simulink model "OTSG_v1"  (R2018a)
settings: Solver=ode23tb  StartTime=0.0  StopTime=2500  MaxStep=0.1  RelTol=1e-3
values from neighbouring files (symbols this model uses):
  A_s = 1.2245    [MSDR_parameters.m]
  Cp_p = 5763.597e-6    (= 0.005763597)    [MSDR_parameters.m]
  Cp_s = 3588.208e-6    (= 0.003588208)    [MSDR_parameters.m]
  Cp_sc = 4761.392e-6    (= 0.004761392)    [MSDR_parameters.m]
  Cp_w = 456.056e-6    (= 0.000456056)    [MSDR_parameters.m]
  D_it = 0.0141478    [MSDR_parameters.m]
  D_ot = 0.015875    [MSDR_parameters.m]
  dHs_dPs = -0.042433622114357    (= -0.0424336221144)    [MSDR_parameters.m]
  h_pw = 9101.343578935E-6    (= 0.00910134357894)    [MSDR_parameters.m]
  h_wb = 13349.334646671E-6    (= 0.0133493346467)    [MSDR_parameters.m]
  h_ws = 5732.378387768E-6    (= 0.00573237838777)    [MSDR_parameters.m]
  h_wsc = 8385.005556375E-6    (= 0.00838500555638)    [MSDR_parameters.m]
  K_1 = 11.632248097704855    (= 11.6322480977)    [MSDR_parameters.m]
  K_b = 12.834854076292217    (= 12.8348540763)    [MSDR_parameters.m]
  K_sc = -17.615718797133468    (= -17.6157187971)    [MSDR_parameters.m]
  L = 8.5344    [MSDR_parameters.m]
  L_b = 5.97408    [MSDR_parameters.m]
  L_s = 1.28016    [MSDR_parameters.m]
  M_stm = 0.018    [MSDR_parameters.m]
  N = 6546    [MSDR_parameters.m]
  P_s = 5.8    [MSDR_parameters.m]
  P_sat = 6    [MSDR_parameters.m]
  P_sc = 5.8    [MSDR_parameters.m]
  P_set = 5.8    [MSDR_parameters.m]
  R = 8.314462E-6    (= 8.314462e-06)    [MSDR_parameters.m]
  rho_p = 716.826    [MSDR_parameters.m]
  rho_s = 26.5561    [MSDR_parameters.m]
  rho_sc = (rho_fw + rho_f)/2    (= 789.7745)    [MSDR_parameters.m]
  rho_w = 8425.712    [MSDR_parameters.m]
  T_p1 = 320.712    [MSDR_parameters.m]
  T_p2 = 320.478    [MSDR_parameters.m]
  T_p3 = 311.033    [MSDR_parameters.m]
  T_p4 = 305.206    [MSDR_parameters.m]
  T_p5 = 303.289    [MSDR_parameters.m]
  T_p6 = 297.506    [MSDR_parameters.m]
  T_s1 = 313.717    [MSDR_parameters.m]
  T_s2 = 307.462    [MSDR_parameters.m]
  T_sc1 = 274.967    [MSDR_parameters.m]
  T_w1 = 320.344    [MSDR_parameters.m]
  T_w2 = 319.794    [MSDR_parameters.m]
  T_w3 = 301.311    [MSDR_parameters.m]
  T_w4 = 299.206    [MSDR_parameters.m]
  T_w5 = 298.512    [MSDR_parameters.m]
  T_w6 = 283.112    [MSDR_parameters.m]
  W_fw = 226.7962    [MSDR_parameters.m]
  W_p0 = 3779.937    [MSDR_parameters.m]
  Z_ss = 0.76634    [MSDR_parameters.m]
settings Model: Creator=viikr  LastModifiedBy=Vikram Singh
settings SolverCC: AlgebraicLoopSolver=LineSearch

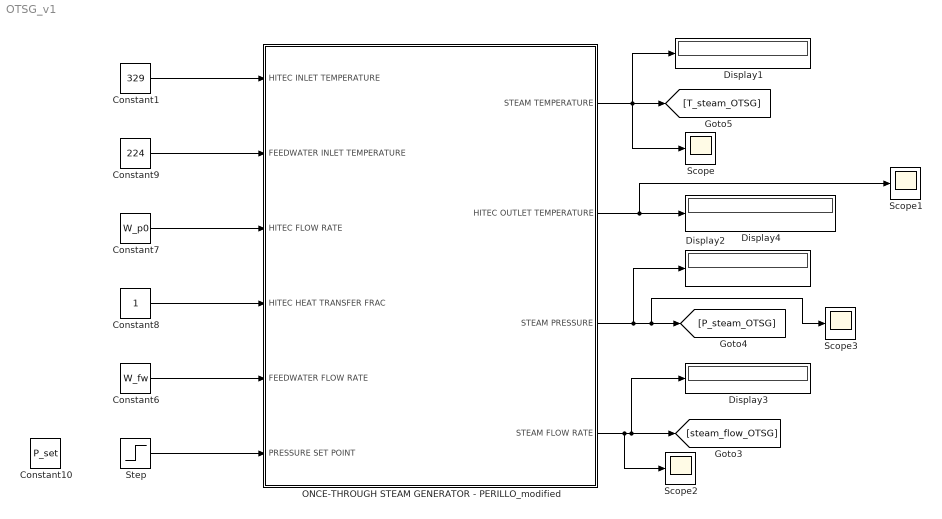
== system OTSG_v1 ==
  Constant1 : Constant  Value=329
  Constant10 : Constant  Value=P_set
  Constant6 : Constant  Value=W_fw
  Constant7 : Constant  Value=W_p0
  Constant8 : Constant
  Constant9 : Constant  Value=224
  Display{1..4} (4 alike) : Display
  ONCE-THROUGH STEAM GENERATOR - PERILLO_modified : Subsystem
  Scope{,1..3} (4 alike) : Scope
  Step : Step  Time=1000  Before=5.8  After=5.9  SampleTime=0
  wires:
  Constant9/1 -> ONCE-THROUGH STEAM GENERATOR - PERILLO_modified/2(FEEDWATER INLET TEMPERATURE)
  ONCE-THROUGH STEAM GENERATOR - PERILLO_modified/1(STEAM TEMPERATURE) -> Scope/1, Display1/1, [T_steam_OTSG]
  Constant8/1 -> ONCE-THROUGH STEAM GENERATOR - PERILLO_modified/4(HITEC HEAT TRANSFER FRAC)
  ONCE-THROUGH STEAM GENERATOR - PERILLO_modified/2(HITEC OUTLET TEMPERATURE) -> Scope1/1, Display4/1
  Constant7/1 -> ONCE-THROUGH STEAM GENERATOR - PERILLO_modified/3(HITEC FLOW RATE)
  ONCE-THROUGH STEAM GENERATOR - PERILLO_modified/4(STEAM FLOW RATE) -> Scope2/1, [steam_flow_OTSG], Display3/1
  ONCE-THROUGH STEAM GENERATOR - PERILLO_modified/3(STEAM PRESSURE) -> Scope3/1, [P_steam_OTSG], Display2/1
  Constant6/1 -> ONCE-THROUGH STEAM GENERATOR - PERILLO_modified/5(FEEDWATER FLOW RATE)
  Constant1/1 -> ONCE-THROUGH STEAM GENERATOR - PERILLO_modified/1(HITEC INLET TEMPERATURE)
  Step/1 -> ONCE-THROUGH STEAM GENERATOR - PERILLO_modified/6(PRESSURE SET POINT)

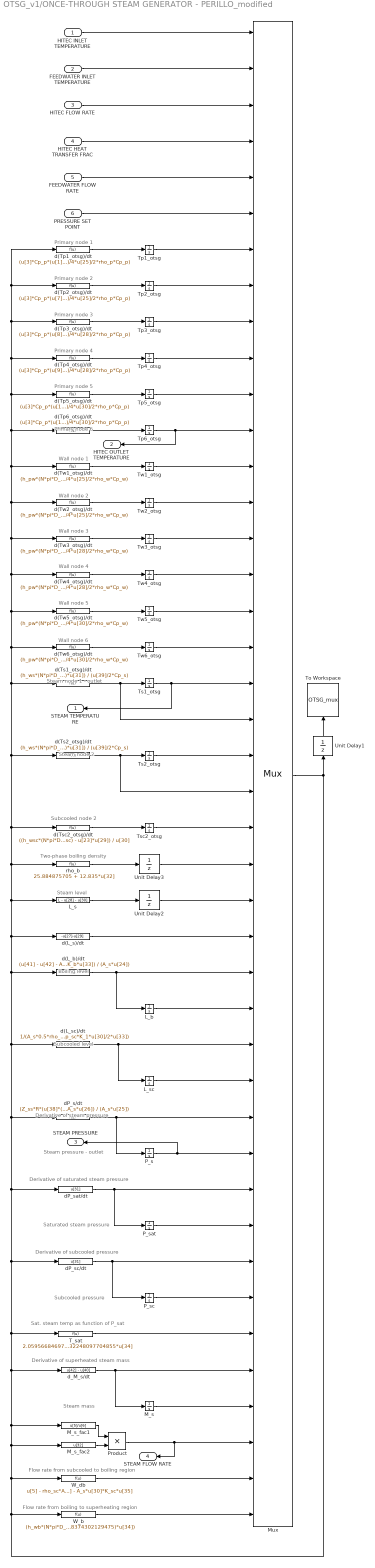
== system OTSG_v1/ONCE-THROUGH STEAM GENERATOR - PERILLO_modified ==
  note: Primary node 1
  note: Primary node 2
  note: Primary node 3
  note: Primary node 4
  note: Primary node 5
  note: Primary node 6
  note: Wall node 1
  note: Wall node 2
  note: Wall node 3
  note: Wall node 4
  note: Wall node 5
  note: Wall node 6
  note: Steam node 1 - outlet
  note: Steam level
  note: Boiling level
  note: Subcooled level
  note: Derivative of saturated steam pressure
  note: Sat. steam temp as function of P_sat
  note: Saturated steam pressure
  note: Subcooled pressure
  note: Derivative of steam pressure
  note: Derivative of subcooled pressure
  note: Steam pressure - outlet
  note: Subcooled node 2
  note: Steam node 2
  note: Two-phase boiling density
  note: Derivative of superheated steam mass
  note: Steam mass
  note: Flow rate from subcooled to boiling region
  note: Flow rate from boiling to superheating region
  HITEC INLET TEMPERATURE : Inport
  FEEDWATER INLET TEMPERATURE : Inport  Port=2
  HITEC FLOW RATE : Inport  Port=3
  HITEC HEAT TRANSFER FRAC : Inport  Port=4
  FEEDWATER FLOW RATE : Inport  Port=5
  PRESSURE SET POINT : Inport  Port=6
  L_b : Integrator  InitialCondition=L_b
  L_s : Fcn  Expr=L - u[28] - u[30]
  L_sc : Integrator  InitialCondition=.5344
  M_s : Integrator  InitialCondition=rho_s*A_s*L_s
  M_s_fac1 : Fcn  Expr=u[5]/u[6]
  M_s_fac2 : Fcn  Expr=u[32]
  Mux : Mux  Inputs=42
      settings: DisplayOption=signals
  P_s : Integrator  InitialCondition=P_s
  P_sat : Integrator  InitialCondition=P_sat
  P_sc : Integrator  InitialCondition=P_sc
  Product : Product
  T_sat : Fcn  Expr=2.059566846979075e+02 + 11.632248097704855*u[34]
  To Workspace : ToWorkspace  VariableName=OTSG_mux  SampleTime=-1
      settings: Save2DSignal=2-D array (concatenate along first dimension)
  Tp1_otsg : Integrator  InitialCondition=T_p1
  Tp2_otsg : Integrator  InitialCondition=T_p2
  Tp3_otsg : Integrator  InitialCondition=T_p3
  Tp4_otsg : Integrator  InitialCondition=T_p4
  Tp5_otsg : Integrator  InitialCondition=T_p5
  Tp6_otsg : Integrator  InitialCondition=T_p6
  Ts1_otsg : Integrator  InitialCondition=T_s1
  Ts2_otsg : Integrator  InitialCondition=T_s2
  Tsc2_otsg : Integrator  InitialCondition=T_sc1
  Tw1_otsg : Integrator  InitialCondition=T_w1
  Tw2_otsg : Integrator  InitialCondition=T_w2
  Tw3_otsg : Integrator  InitialCondition=T_w3
  Tw4_otsg : Integrator  InitialCondition=T_w4
  Tw5_otsg : Integrator  InitialCondition=T_w5
  Tw6_otsg : Integrator  InitialCondition=T_w6
  Unit Delay1 : UnitDelay  SampleTime=-1
  Unit Delay2 : UnitDelay  InitialCondition=L_s  SampleTime=-1
  Unit Delay3 : UnitDelay  InitialCondition=100.307656893  SampleTime=-1
  W_b : Fcn  Expr=(h_wb*(N*pi*D_ot*u[28])*(0.5*u[15] + 0.5*u[16] - u[37])) / (1.980883222760319 + (-0.068374302129475)*u[34])
  W_db : Fcn  Expr=u[5] - rho_sc*A_s*u[29] - A_s*u[30]*K_sc*u[35]
  d(L_b)/dt : Fcn  Expr=(u[41] - u[42] - A_s*u[28]*K_b*u[33]) / (A_s*u[24])
  d(L_s)/dt : Fcn  Expr=-u[27]-u[29]
  d(L_sc)/dt : Fcn  Expr=1/(A_s*0.5*rho_sc*Cp_sc*(u[23] - u[37])) * (h_wsc*N*pi*D_ot*u[30]/2*(u[17] - u[37]) + u[5]*Cp_sc*(u[23] - u[37]) - A_s*u[30]/2*(K_sc*Cp_sc*(u[23] - 2*u[37]) - 1)*u[35] - A_s*rho_sc*Cp_sc*K_1*u[30]/2*u[33])
  d(Tp1_otsg)/dt : Fcn  Expr=(u[3]*Cp_p*(u[1] - u[7]) + h_pw*(N*pi*D_it*u[25]/2)*(u[13] - u[7])) / (N*pi*(D_it^2)/4*u[25]/2*rho_p*Cp_p)
  d(Tp2_otsg)/dt : Fcn  Expr=(u[3]*Cp_p*(u[7] - u[8]) + h_pw*(N*pi*D_it*u[25]/2)*(u[14] - u[8])) / (N*pi*(D_it^2)/4*u[25]/2*rho_p*Cp_p)
  d(Tp3_otsg)/dt : Fcn  Expr=(u[3]*Cp_p*(u[8] - u[9]) + h_pw*(N*pi*D_it*u[28]/2)*(u[15] - u[9])) / (N*pi*(D_it^2)/4*u[28]/2*rho_p*Cp_p)
  d(Tp4_otsg)/dt : Fcn  Expr=(u[3]*Cp_p*(u[9] - u[10]) + h_pw*(N*pi*D_it*u[28]/2)*(u[16] - u[10])) / (N*pi*(D_it^2)/4*u[28]/2*rho_p*Cp_p)
  d(Tp5_otsg)/dt : Fcn  Expr=(u[3]*Cp_p*(u[10] - u[11]) + h_pw*(N*pi*D_it*u[30]/2)*(u[17] - u[11])) / (N*pi*(D_it^2)/4*u[30]/2*rho_p*Cp_p)
  d(Tp6_otsg)/dt : Fcn  Expr=(u[3]*Cp_p*(u[11] - u[12]) + h_pw*(N*pi*D_it*u[30]/2)*(u[18] - u[12])) / (N*pi*(D_it^2)/4*u[30]/2*rho_p*Cp_p)
  d(Ts1_otsg)/dt : Fcn  Expr=(h_ws*(N*pi*D_ot*u[25]/2)*(u[13] - u[19]) + u[40]*Cp_s*(u[21] - u[19]) + Cp_s*(u[21] - u[19])*u[38]/2 + (A_s*u[25]/2 - u[39]/2*dHs_dPs)*u[31]) / (u[39]/2*Cp_s)
  d(Ts2_otsg)/dt : Fcn  Expr=(h_ws*(N*pi*D_ot*u[25]/2)*(u[14] - u[21]) + u[42]*Cp_s*(u[37] - u[21]) + (A_s*u[25]/2 - u[39]/2*dHs_dPs)*u[31]) / (u[39]/2*Cp_s)
  d(Tsc2_otsg)/dt : Fcn  Expr=((h_wsc*(N*pi*D_ot*u[30]/2)*(u[18] - u[23]) + Cp_sc*(u[5]*u[2] - (u[5] + u[41])*0.5*u[23]) + A_s*u[30]/2*u[35]) * 2/(A_s*rho_sc*Cp_sc) - u[23]*u[29]) / u[30]
  d(Tw1_otsg)/dt : Fcn  Expr=(h_pw*(N*pi*D_it*u[25]/2)*(u[7] - u[13]) + h_ws*(N*pi*D_ot*u[25]/2)*(u[19] - u[13])) / (N*pi*(D_ot^2 - D_it^2)/4*u[25]/2*rho_w*Cp_w)
  d(Tw2_otsg)/dt : Fcn  Expr=(h_pw*(N*pi*D_it*u[25]/2)*(u[8] - u[14]) + h_ws*(N*pi*D_ot*u[25]/2)*(u[21] - u[14])) / (N*pi*(D_ot^2 - D_it^2)/4*u[25]/2*rho_w*Cp_w)
  d(Tw3_otsg)/dt : Fcn  Expr=(h_pw*(N*pi*D_it*u[28]/2)*(u[9] - u[15]) + h_wb*(N*pi*D_ot*u[28]/2)*(u[37] - u[15])) / (N*pi*(D_ot^2 - D_it^2)/4*u[28]/2*rho_w*Cp_w)
  d(Tw4_otsg)/dt : Fcn  Expr=(h_pw*(N*pi*D_it*u[28]/2)*(u[10] - u[16]) + h_wb*(N*pi*D_ot*u[28]/2)*(u[37] - u[16])) / (N*pi*(D_ot^2 - D_it^2)/4*u[28]/2*rho_w*Cp_w)
  d(Tw5_otsg)/dt : Fcn  Expr=(h_pw*(N*pi*D_it*u[30]/2)*(u[11] - u[17]) + h_wsc*(N*pi*D_ot*u[30]/2)*(u[37] - u[17])) / (N*pi*(D_ot^2 - D_it^2)/4*u[30]/2*rho_w*Cp_w)
  d(Tw6_otsg)/dt : Fcn  Expr=(h_pw*(N*pi*D_it*u[30]/2)*(u[12] - u[18]) + h_wsc*(N*pi*D_ot*u[30]/2)*(u[23] - u[18])) / (N*pi*(D_ot^2 - D_it^2)/4*u[30]/2*rho_w*Cp_w)
  dP_s/dt : Fcn  Expr=(Z_ss*R*(u[38]*(u[19] + u[21]) + u[39]*(u[20] + u[22]))/(2*M_stm) - u[32]*A_s*u[26]) / (A_s*u[25])
  dP_sat/dt : Fcn  Expr=u[31]
  dP_sc/dt : Fcn  Expr=u[31]
  d_M_s/dt : Fcn  Expr=u[42] - u[40]
  rho_b : Fcn  Expr=25.884875705 + 12.835*u[32]
  STEAM TEMPERATURE : Outport
  HITEC OUTLET TEMPERATURE : Outport  Port=2
  STEAM PRESSURE : Outport  Port=3
  STEAM FLOW RATE : Outport  Port=4
  wires:
  FEEDWATER INLET TEMPERATURE/1 -> Mux/2
  d(Tp1_otsg)/dt/1 -> Tp1_otsg/1
  HITEC INLET TEMPERATURE/1 -> Mux/1
  HITEC FLOW RATE/1 -> Mux/3
  HITEC HEAT TRANSFER FRAC/1 -> Mux/4
  FEEDWATER FLOW RATE/1 -> Mux/5
  PRESSURE SET POINT/1 -> Mux/6
  Tp1_otsg/1 -> Mux/7
  Tp2_otsg/1 -> Mux/8
  d(Tp2_otsg)/dt/1 -> Tp2_otsg/1
  Tp3_otsg/1 -> Mux/9
  d(Tp3_otsg)/dt/1 -> Tp3_otsg/1
  Tp4_otsg/1 -> Mux/10
  d(Tp4_otsg)/dt/1 -> Tp4_otsg/1
  Tp5_otsg/1 -> Mux/11
  d(Tp5_otsg)/dt/1 -> Tp5_otsg/1
  d(Tp6_otsg)/dt/1 -> Tp6_otsg/1
  Tp6_otsg/1 -> HITEC OUTLET TEMPERATURE/1, Mux/12
  Tw1_otsg/1 -> Mux/13
  d(Tw1_otsg)/dt/1 -> Tw1_otsg/1
  d(Tw2_otsg)/dt/1 -> Tw2_otsg/1
  Tw2_otsg/1 -> Mux/14
  Tw3_otsg/1 -> Mux/15
  d(Tw3_otsg)/dt/1 -> Tw3_otsg/1
  d(Tw4_otsg)/dt/1 -> Tw4_otsg/1
  Tw4_otsg/1 -> Mux/16
  Tw5_otsg/1 -> Mux/17
  d(Tw5_otsg)/dt/1 -> Tw5_otsg/1
  d(Tw6_otsg)/dt/1 -> Tw6_otsg/1
  Tw6_otsg/1 -> Mux/18
  Ts1_otsg/1 -> STEAM TEMPERATURE/1, Mux/19
  L_sc/1 -> Mux/30
  L_s/1 -> Unit Delay2/1
  d(L_s)/dt/1 -> Mux/26
  Unit Delay2/1 -> Mux/25
  L_b/1 -> Mux/28
  dP_sc/dt/1 -> Mux/35, P_sc/1
  P_s/1 -> Mux/32, STEAM PRESSURE/1
  P_sat/1 -> Mux/34
  P_sc/1 -> Mux/36
  dP_sat/dt/1 -> Mux/33, P_sat/1
  T_sat/1 -> Mux/37
  dP_s/dt/1 -> Mux/31, P_s/1
  Tsc2_otsg/1 -> Mux/23
  d(Tsc2_otsg)/dt/1 -> Tsc2_otsg/1
  Ts2_otsg/1 -> Mux/21
  rho_b/1 -> Unit Delay3/1
  Unit Delay3/1 -> Mux/24
  d(Ts1_otsg)/dt/1 -> Mux/20, Ts1_otsg/1
  d(Ts2_otsg)/dt/1 -> Mux/22, Ts2_otsg/1
  M_s/1 -> Mux/39
  d_M_s/dt/1 -> Mux/38, M_s/1
  M_s_fac1/1 -> Product/1
  M_s_fac2/1 -> Product/2
  W_db/1 -> Mux/41
  d(L_b)/dt/1 -> Mux/27, L_b/1
  d(L_sc)/dt/1 -> Mux/29, L_sc/1
  Mux/1 -> Unit Delay1/1, W_b/1, W_db/1, M_s_fac2/1, d_M_s/dt/1, T_sat/1, dP_sc/dt/1, dP_sat/dt/1, dP_s/dt/1, d(L_sc)/dt/1, d(L_b)/dt/1, d(L_s)/dt/1, L_s/1, rho_b/1, d(Tsc2_otsg)/dt/1, d(Ts2_otsg)/dt/1, d(Ts1_otsg)/dt/1, d(Tw6_otsg)/dt/1, d(Tw5_otsg)/dt/1, d(Tw4_otsg)/dt/1, d(Tw3_otsg)/dt/1, d(Tw2_otsg)/dt/1, d(Tw1_otsg)/dt/1, d(Tp6_otsg)/dt/1, d(Tp5_otsg)/dt/1, d(Tp4_otsg)/dt/1, d(Tp3_otsg)/dt/1, d(Tp2_otsg)/dt/1, d(Tp1_otsg)/dt/1, M_s_fac1/1
  W_b/1 -> Mux/42
  Product/1 -> Mux/40, STEAM FLOW RATE/1
  Unit Delay1/1 -> To Workspace/1
